simulink model "turbinedcc"  (R2022b)
settings: Solver=VariableStepAuto  StartTime=0.0  StopTime=10.0  RelTol=1e-3
undefined symbols (not defined in the file): DiscIntNeverNeededParam, Ion, Lithium
libraries: spsDiodeLib x7, spsVoltageMeasurementLib x5, spsSeriesRLCBranchLib x4, spsCurrentMeasurementLib x3, spsRMSLib x2, spsBatteryLib x1, spsFirstOrderFilterLib x1, spsPWMGeneratorDCDCLib x1, spsPermanentMagnetSynchronousMachineLib x1, spsIGBTDiodeLib x1, spsThreePhaseVIMeasurementLib x1, spsWindTurbineLib x1
settings Model: Creator=CC  LastModifiedBy=admin
settings SolverCC: AlgebraicLoopSolver=TrustRegion
settings DataIOCC: ReturnWorkspaceOutputs=off
settings DebuggingCC: UnconnectedInputMsg=warning  UnconnectedOutputMsg=warning  UnconnectedLineMsg=warning  SFMachineParentedDataDiag=warning  ArithmeticOperatorsInVariantConditions=warning
settings ModelReferenceCC: EnableRefExpFcnMdlSchedulingChecks=on
settings SFSimCC: SimUseLocalCustomCode=off  CustomCodeUndefinedFunction=UseInterfaceOnly
settings RTWCC: RTWUseLocalCustomCode=off

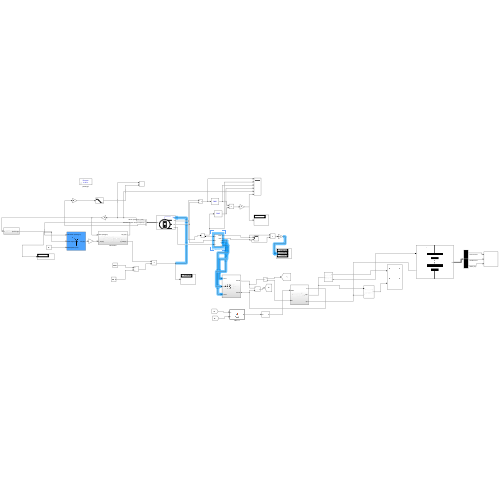
[thumbnail: Simulink's stored preview of the top-level diagram]
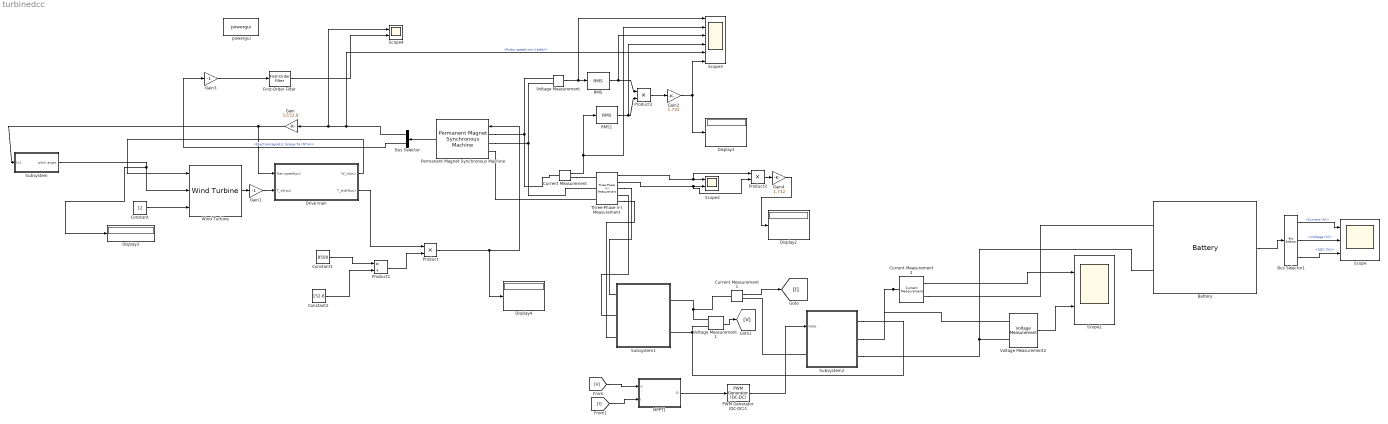
== system turbinedcc ==
  Battery : spsBatteryLib/Battery  BatType=Lithium-Ion  ShowTempParam=off  ThermalPreset=no  ShowAgeParam=off  NomV=7.2  NomQ=5.4  SOC=25  Batt_Tr=30  PresetModel=off  MaxQ=5.4  MinV=5.4  FullV=8.3807  Dis_rate=2.3478  R=0.013333  Normal_OP=4.8835  expZone="[7.7788      0.2653]"  current=[6.5 13 32.5]  Units=Time  Tci=20  NomT=20  T2=-30  MaxQ2=4.8  FullV2=7.1  Normal_OP2=5.655  expZone2="[6.58           1]"  Rca=0.6  ti=2000  Dp=0  Neq0=0  Tsim=1e6  Ta1=25  Qeol=5.4*0.9  Reol=0.013333*1.2  Char_age=[2.3478, 3]  Dis_age=[2.3478, 10]  N1=1500  N2=10500  N3=1000  N4=1400  Ta2=45  N5=950
      settings: LibrarySourceBlock=electricdrivelib/Extra Sources/Battery
  Bus Selector : BusSelector  OutputSignals=Rotor speed wm (rad/s),Electromagnetic torque Te (N*m)
  Bus Selector1 : BusSelector  OutputSignals=Current (A),Voltage (V),SOC (%)
  Constant : Constant  Value=12
  Constant1 : Constant  Value=8500
  Constant2 : Constant  Value=152.8
  Current Measurement : spsCurrentMeasurementLib/Current Measurement  PhasorSimulation=off  OutputType=Complex  PSBequivalent=0
  Current Measurement1 : spsCurrentMeasurementLib/Current Measurement  PhasorSimulation=off  OutputType=Complex  PSBequivalent=0
  Current Measurement2 : spsCurrentMeasurementLib/Current Measurement  PhasorSimulation=off  OutputType=Complex  PSBequivalent=0
  Display{1..4} (4 alike) : Display
  "Drive train " : Subsystem
  First-Order Filter : spsFirstOrderFilterLib/First-Order Filter  FilterType=Lowpass  Tc=1e-3  Ts=50e-6  Initialize=on  Vac_Init=[0, 0, 50]  Vdc_Init=0  PlotResponse=off  FreqRange="[0,  200,  1]"
  Gain : Gain  Gain=1/152.8
  Gain1 : Gain  Gain=-1
  Gain2 : Gain  Gain=1.732
  Gain3 : Gain  Gain=-1
  Gain4 : Gain  Gain=1.732
  MPPT1 : MATLAB Function  TreatAsAtomicUnit=on
  PWM Generator (DC-DC)1 : spsPWMGeneratorDCDCLib/PWM Generator (DC-DC)  Fsw=5000  Ts=10e-6
  Permanent Magnet Synchronous Machine : spsPermanentMagnetSynchronousMachineLib/Permanent Magnet Synchronous Machine  NbPhases=3  FluxDistribution=Sinusoidal  RotorType=Round  MechanicalLoad=Torque Tm  PresetModel=No  ShowDetailedParameters=on  MeasurementBus=off  Resistance=0.425  Inductance=8.5e-3  dqInductances=[8.5e-3,8.5e-3]  La=0.000395  MachineConstant=Flux linkage established by magnets (V.s)  Flux=0.433  VoltageCst=392.6876  TorqueCst=3.2475  Flat=120  Mechanical=[0.01197 0.001189 5 0]  PolePairs=4  InitialConditions=[0,0, 0,0]  InitialConditions5ph=[0 0 0 0 0 0]  RefAngle=90 degrees behind phase A axis (modified Park)  IterativeDiscreteModel=Trapezoidal non iterative  TsBlock=-1  TsPowergui=0
  Product : Product
  Product1 : Product  Inputs=*/
  Product2 : Product
  Product3 : Product
  RMS : spsRMSLib/RMS  TrueRMS=on  Freq=50  RMSInit=120  Ts=50e-6
  RMS1 : spsRMSLib/RMS  TrueRMS=on  Freq=50  RMSInit=120  Ts=50e-6
  Scope : Scope  NumInputPorts=3
  Scope1 : Scope  NumInputPorts=2
  Scope2 : Scope  NumInputPorts=2
  Scope3 : Scope  NumInputPorts=6
  Scope4 : Scope  NumInputPorts=2
  Subsystem : Subsystem
  Subsystem1 : Subsystem
  Subsystem2 : Subsystem
  Three-Phase V-I Measurement : spsThreePhaseVIMeasurementLib/Three-Phase V-I Measurement  VoltageMeasurement=phase-to-phase  SetLabelV=off  LabelV=Vabc  Vpu=off  VpuLL=off  CurrentMeasurement=yes  SetLabelI=off  LabelI=Iabc  Ipu=off  Pbase=100e6  Vbase=500e3  OutputType=Complex  PhasorSimulation=off  PSBequivalent=0
  Voltage Measurement : spsVoltageMeasurementLib/Voltage Measurement  PhasorSimulation=off  OutputType=Complex  PSBequivalent=0
  Voltage Measurement1 : spsVoltageMeasurementLib/Voltage Measurement  PhasorSimulation=off  OutputType=Complex  PSBequivalent=0
  Voltage Measurement2 : spsVoltageMeasurementLib/Voltage Measurement  PhasorSimulation=off  OutputType=Complex  PSBequivalent=0
  Wind Turbine : spsWindTurbineLib/Wind Turbine  Pnom=8.5e3  Pelec_base=8.5e3/0.9  wind_base=12  P_wind_base=0.8  speed_nom=1  pitch_angle=0  c1_c6="[0.51763          116          0.4            5           21     0.006795]"  cp_nom=0.48  lambda_nom=8.1
  powergui : sps_lib/powergui  Priority=1  SimulationMode=Discrete  SampleTime=1e-6  frequency=60  Iterations=50  frequencyindice=0  Pbase=100e6  ErrMax=1e-4  UnitsV=kV  UnitsW=MW  buscounter=0  FunctionMessages=off  echomessages=off  EnableUseOfTLC=off  CurrentSourceSwitches=off  DisableSnubberDevices=off  DisableRonSwitches=off  DisableVfSwitches=off  DisplayEquations=off  AutomaticDiscreteSolvers=off  SolverType=Tustin/Backward Euler (TBE)  Interpol=off  ExternalGateDelay=off  methode=off  Ts=100  x0status=blocks  SPID=on  SwTol=0  HookPort=off  NonlinearTolerance=1e-4  nMaxIteration=100  ContinueOnMaxIteration=off  RestoreLinks=warning  ResistiveCurrentMeasurement=off  Frange=[0:2:500]  Ylog=off  Xlog=on  ShowGrid=off  save=off  variable=ZData  structure=0  ZoomFFT=off  StartTime=0.0  cycles=1  DisplayStyle=1  fundamental=60  FreqAxis=off  MaxFrequency=1000  frequencyindicesteady=1  RmsSteady=1  display=off
  wires:
  Product2/1 -> Gain2/1
  Constant/1 -> Wind Turbine/3
  Three-Phase V-I Measurement/1 -> Product3/1, Scope2/1
  First-Order Filter/1 -> Scope4/2
  Permanent Magnet Synchronous Machine/1 -> Bus Selector/1
  RMS1/1 -> Scope3/4, Product2/2
  Gain2/1 -> Scope3/6, Display1/1
  Constant1/1 -> Product1/1
  Three-Phase V-I Measurement/2 -> Product3/2, Scope2/2
  Subsystem/1(pitch angle) -> Display3/1, Wind Turbine/2
  Current Measurement/1 -> Scope3/2, RMS1/1
  Gain1/1 -> "Drive train "/2(T_wt(pu))
  "Drive train "/2(T_shaft(pu)) -> Product/1
  Product/1 -> Display4/1, Permanent Magnet Synchronous Machine/1
  Bus Selector/2 -> Gain3/1  "<Electromagnetic torque Te (N*m)>"
  Gain3/1 -> First-Order Filter/1
  Voltage Measurement/1 -> Scope3/1, RMS/1
  "Drive train "/1(W_w(pu)) -> Wind Turbine/1
  Product1/1 -> Product/2
  Constant2/1 -> Product1/2
  Gain/1 -> Subsystem/1(In1), "Drive train "/1(Gen speed(pu))
  RMS/1 -> Scope3/3, Product2/1
  Bus Selector/1 -> Scope3/5, Scope4/1, Gain/1  "<Rotor speed wm (rad/s)>"
  Wind Turbine/1 -> Gain1/1
  Product3/1 -> Gain4/1
  Gain4/1 -> Display2/1
  Bus Selector1/3 -> Scope/3  "<SOC (%)>"
  Bus Selector1/1 -> Scope/1  "<Current (A)>"
  Bus Selector1/2 -> Scope/2  "<Voltage (V)>"
  Voltage Measurement2/1 -> Scope1/2
  Battery/1 -> Bus Selector1/1
  [I] -> MPPT1/2(I)
  Current Measurement1/1 -> [I]
  [V] -> MPPT1/1(V)
  Current Measurement2/1 -> Scope1/1
  MPPT1/1(D) -> PWM Generator (DC-DC)1/1
  Voltage Measurement1/1 -> [V]
  PWM Generator (DC-DC)1/1 -> Subsystem2/1(Gate)
  connections:
  Voltage Measurement/LConn2 -- Permanent Magnet Synchronous Machine/LConn2 -- Three-Phase V-I Measurement/LConn2
  Voltage Measurement/LConn1 -- Permanent Magnet Synchronous Machine/LConn1 -- Current Measurement/LConn1
  Three-Phase V-I Measurement/RConn3 -- Subsystem1/RConn3
  Permanent Magnet Synchronous Machine/LConn3 -- Three-Phase V-I Measurement/LConn3
  Subsystem1/RConn2 -- Three-Phase V-I Measurement/RConn2
  Current Measurement/RConn1 -- Three-Phase V-I Measurement/LConn1
  Three-Phase V-I Measurement/RConn1 -- Subsystem1/RConn1
  Voltage Measurement2/LConn2 -- Subsystem2/RConn3 -- Battery/LConn2
  Subsystem2/RConn1 -- Subsystem1/LConn2 -- Voltage Measurement1/LConn2
  Current Measurement1/LConn1 -- Voltage Measurement1/LConn1 -- Subsystem1/LConn1
  Current Measurement2/LConn1 -- Subsystem2/RConn2 -- Voltage Measurement2/LConn1
  Current Measurement2/RConn1 -- Battery/LConn1
  Subsystem2/LConn1 -- Current Measurement1/RConn1

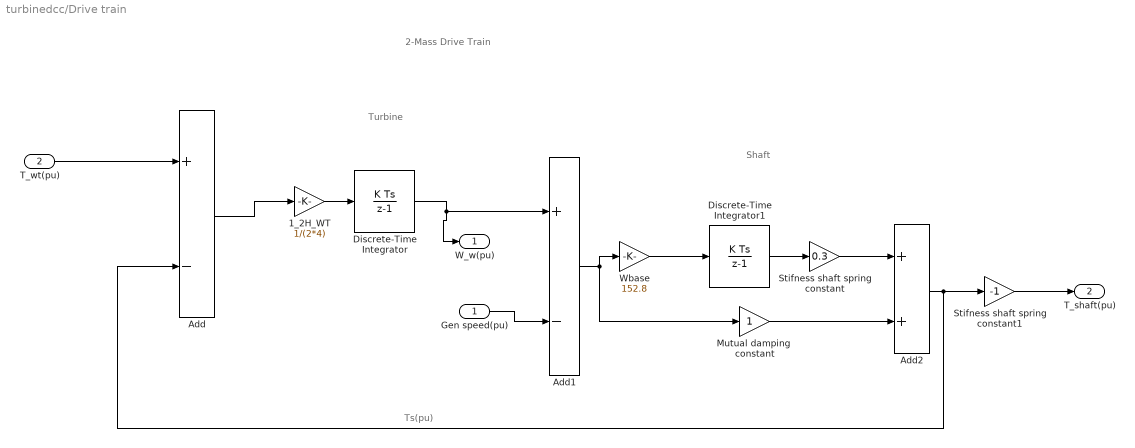
== system turbinedcc/Drive train  ==
  note: Shaft
  note: Turbine
  note: 2-Mass Drive Train
  note: Ts(pu)
  Gen speed(pu) : Inport
  T_wt(pu) : Inport  Port=2
  1_2H_WT : Gain  Gain=1/(2*4)
  Add : Sum  Inputs=+-
  Add1 : Sum  Inputs=+-
  Add2 : Sum
  Discrete-Time Integrator : DiscreteIntegrator  InitialCondition=1  SampleTime=50e-6  ICPrevOutput=DiscIntNeverNeededParam  ICPrevScaledInput=DiscIntNeverNeededParam
  Discrete-Time Integrator1 : DiscreteIntegrator  InitialCondition=1/0.3  SampleTime=50e-6  ICPrevOutput=DiscIntNeverNeededParam  ICPrevScaledInput=DiscIntNeverNeededParam
  Mutual damping  constant : Gain
  Stifness shaft spring constant : Gain  Gain=0.3
  Stifness shaft spring constant1 : Gain  Gain=-1
  Wbase : Gain  Gain=152.8
  W_w(pu) : Outport  VectorParamsAs1DForOutWhenUnconnected=off
  T_shaft(pu) : Outport  Port=2  VectorParamsAs1DForOutWhenUnconnected=off
  wires:
  T_wt(pu)/1 -> Add/1
  Add/1 -> 1_2H_WT/1
  1_2H_WT/1 -> Discrete-Time Integrator/1
  Discrete-Time Integrator/1 -> W_w(pu)/1, Add1/1
  Gen speed(pu)/1 -> Add1/2
  Add1/1 -> Wbase/1, Mutual damping  constant/1
  Wbase/1 -> Discrete-Time Integrator1/1
  Discrete-Time Integrator1/1 -> Stifness shaft spring constant/1
  Stifness shaft spring constant/1 -> Add2/1
  Mutual damping  constant/1 -> Add2/2
  Add2/1 -> Stifness shaft spring constant1/1, Add/2
  Stifness shaft spring constant1/1 -> T_shaft(pu)/1

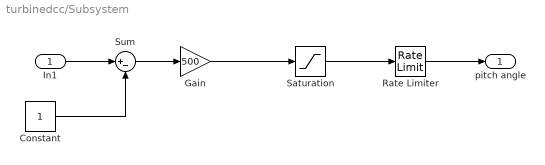
== system turbinedcc/Subsystem ==
  In1 : Inport
  Constant : Constant
  Gain : Gain  Gain=500
  Rate Limiter : RateLimiter  RisingSlewLimit=2  FallingSlewLimit=-2  SampleTimeMode=inherited
  Saturation : Saturate  UpperLimit=45  LowerLimit=0  ZeroCross=off
  Sum : Sum  Inputs=|+-
  pitch angle : Outport  VectorParamsAs1DForOutWhenUnconnected=off
  wires:
  In1/1 -> Sum/1
  Constant/1 -> Sum/2
  Sum/1 -> Gain/1
  Gain/1 -> Saturation/1
  Saturation/1 -> Rate Limiter/1
  Rate Limiter/1 -> pitch angle/1

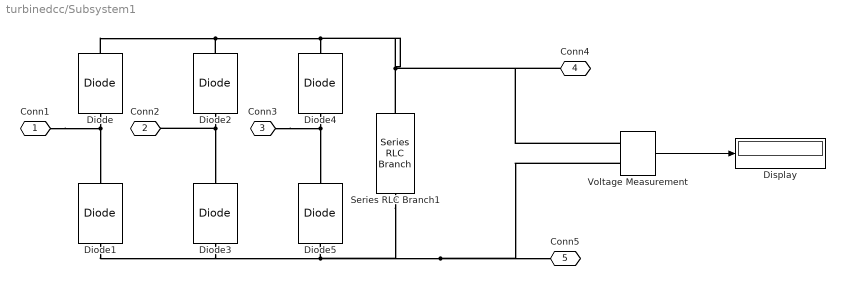
== system turbinedcc/Subsystem1 ==
  Diode{,1..5} (6 alike) : spsDiodeLib/Diode  Ron=0.001  Lon=0  Vf=0.8  IC=0  UseSnubber=0  Rs=500  Cs=250e-9  Measurements=off
  Display : Display
  Series RLC Branch1 : spsSeriesRLCBranchLib/Series RLC Branch  LConnTagsString=__new0  RConnTagsString=__new0  BranchType=C  Resistance=10  Inductance=1e-3  SetiL0=off  InitialCurrent=0  Capacitance=10e-3  Setx0=off  InitialVoltage=0  Measurements=Branch current
  Voltage Measurement : spsVoltageMeasurementLib/Voltage Measurement  PhasorSimulation=off  OutputType=Complex  PSBequivalent=0
  Conn1 : PMIOPort  Side=Right
  Conn2 : PMIOPort  Port=2  Side=Right
  Conn3 : PMIOPort  Port=3  Side=Right
  Conn4 : PMIOPort  Port=4  Side=Left
  Conn5 : PMIOPort  Port=5  Side=Left
  wires:
  Voltage Measurement/1 -> Display/1
  connections:
  Diode5/LConn1 -- Diode1/LConn1 -- Diode3/LConn1 -- Series RLC Branch1/LConn1 -- Voltage Measurement/LConn2 -- Conn5/RConn1
  Diode4/LConn1 -- Conn3/RConn1 -- Diode5/RConn1
  Diode/RConn1 -- Diode2/RConn1 -- Diode4/RConn1 -- Series RLC Branch1/RConn1 -- Conn4/RConn1 -- Voltage Measurement/LConn1
  Diode2/LConn1 -- Conn2/RConn1 -- Diode3/RConn1
  Diode/LConn1 -- Conn1/RConn1 -- Diode1/RConn1

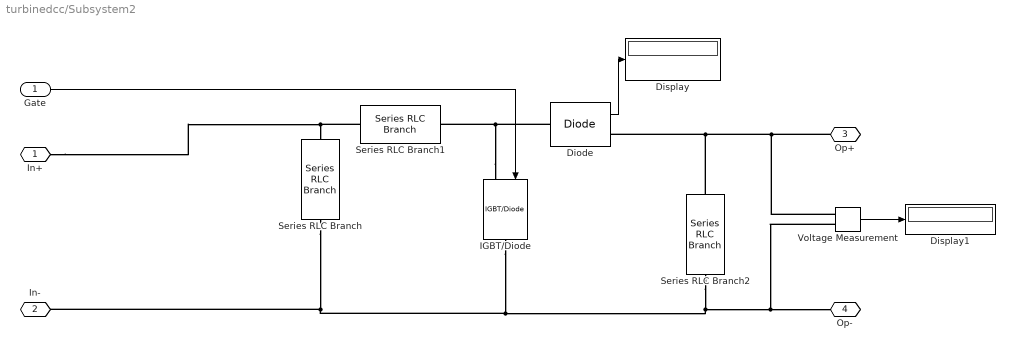
== system turbinedcc/Subsystem2 ==
  Gate : Inport
  Diode : spsDiodeLib/Diode  Ron=0.001  Lon=0  Vf=0.8  IC=0  UseSnubber=0  Rs=500  Cs=250e-9  Measurements=on
  Display : Display
  Display1 : Display
  IGBT/Diode : spsIGBTDiodeLib/IGBT//Diode  Ron=1e-3  Rs=1e5  Cs=inf  Measurements=off
  Series RLC Branch : spsSeriesRLCBranchLib/Series RLC Branch  LConnTagsString=__new0  RConnTagsString=__new0  BranchType=RC  Resistance=1e-4  Inductance=1e-3  SetiL0=off  InitialCurrent=0  Capacitance=100e-6  Setx0=off  InitialVoltage=0  Measurements=None
  Series RLC Branch1 : spsSeriesRLCBranchLib/Series RLC Branch  LConnTagsString=__new0  RConnTagsString=__new0  BranchType=RL  Resistance=0.1  Inductance=5e-3  SetiL0=off  InitialCurrent=0  Capacitance=100e-6  Setx0=off  InitialVoltage=0  Measurements=None
  Series RLC Branch2 : spsSeriesRLCBranchLib/Series RLC Branch  LConnTagsString=__new0  RConnTagsString=__new0  BranchType=RC  Resistance=1e-4  Inductance=1e-3  SetiL0=off  InitialCurrent=0  Capacitance=3300e-6  Setx0=off  InitialVoltage=0  Measurements=None
  Voltage Measurement : spsVoltageMeasurementLib/Voltage Measurement  PhasorSimulation=off  OutputType=Complex  PSBequivalent=0
  In+ : PMIOPort  Side=Left
  In- : PMIOPort  Port=2  Side=Right
  Op+ : PMIOPort  Port=3  Side=Right
  Op- : PMIOPort  Port=4  Side=Right
  wires:
  Diode/1 -> Display/1
  Gate/1 -> IGBT/Diode/1
  Voltage Measurement/1 -> Display1/1
  connections:
  IGBT/Diode/LConn1 -- Series RLC Branch1/RConn1 -- Diode/LConn1
  Voltage Measurement/LConn2 -- IGBT/Diode/RConn1 -- Series RLC Branch/RConn1 -- In-/RConn1 -- Series RLC Branch2/RConn1 -- Op-/RConn1
  Series RLC Branch2/LConn1 -- Diode/RConn1 -- Op+/RConn1 -- Voltage Measurement/LConn1
  Series RLC Branch1/LConn1 -- Series RLC Branch/LConn1 -- In+/RConn1

== matlab function turbinedcc/MPPT1 ==
  data: V input; D output; I input
function D = Pand0(V,I)

Dinit = 0.39;    %Initial value for D output


persistent Dprev Pprev Vprev

if isempty (Dprev) 
   
Dprev = Dinit;

Vprev = 0;

Pprev = 0;

end

deltaD = 125e-6;

% Calculate measured array power

P = V*I;

% Increase or decrease duty cycle based on conditions

if (P-Pprev) ~= 0 
    if (P-Pprev) > 0

if (V-Vprev) > 0

D= Dprev - deltaD;

else

D = Dprev + deltaD;

end

else

if (V-Vprev) > 0

D= Dprev + deltaD;

else

D = Dprev - deltaD;

end
    end
else
    D = Dprev;
end
% Update internal values

Dprev = D;

Vprev = V; 

Pprev = P;
